simulink model "orbit_propagator"  (R2023b)
settings: Solver=VariableStepAuto  StartTime=0.0  StopTime=10.0  RelTol=1e-3
settings Model: Creator=annahylbert  LastModifiedBy=annahylbert

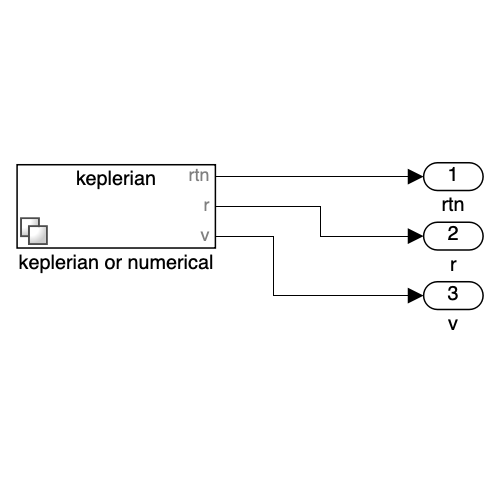
[thumbnail: Simulink's stored preview of the top-level diagram]
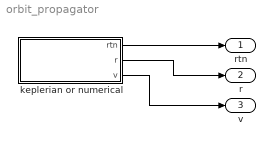
== system orbit_propagator ==
  keplerian or numerical : Subsystem  Variant=on
  rtn : Outport
  r : Outport  Port=2
  v : Outport  Port=3
  wires:
  keplerian or numerical/1(rtn) -> rtn/1
  keplerian or numerical/2(r) -> r/1
  keplerian or numerical/3(v) -> v/1

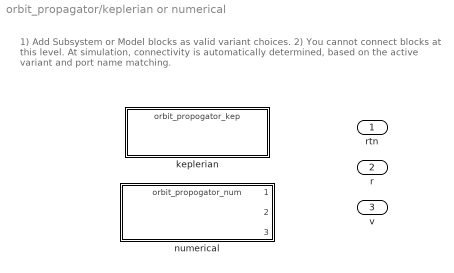
== system orbit_propagator/keplerian or numerical ==
  note: 1) Add Subsystem or Model blocks as valid variant choices.
      | 2) You cannot connect blocks at this level. At simulation, connectivity is automatically
      | determined, based on the active variant and port name matching.
  keplerian : ModelReference  ModelNameDialog=orbit_propogator_kep.slx  SimulationMode=Normal  VariantControl="orbitType==\"kep\""  ModelReferenceVersion=1.19
  numerical : ModelReference  ModelNameDialog=orbit_propogator_num.slx  SimulationMode=Normal  VariantControl="orbitType==\"num\""  ModelReferenceVersion=1.24
  rtn : Outport
  r : Outport  Port=2
  v : Outport  Port=3
